simulink model "Q3"  (R2021b)
settings: Solver=ode45  StartTime=0.0  StopTime=30  RelTol=1e-3  EnableMultiTasking=on
undefined symbols (not defined in the file or in its folder): Hds, Hfs, Hus, V_s, Vs_nd
settings Model: Creator=ak  LastModifiedBy=user
settings SolverCC: AlgebraicLoopSolver=TrustRegion
settings DataIOCC: LimitDataPoints=on  SaveFormat=Array  ReturnWorkspaceOutputs=off
settings OptimizationCC: ExpressionDepthLimit=2147483647  LifeSpan=inf
settings DebuggingCC: UnderspecifiedInitializationDetection=Classic  MergeDetectMultiDrivingBlocksExec=none  SolverPrmCheckMsg=warning  StateNameClashWarn=warning  SFUnexpectedBacktrackingDiag=warning  SFNoUnconditionalDefaultTransitionDiag=warning  SFExecutionAtInitializationDiag=none  SFMachineParentedDataDiag=warning  ArithmeticOperatorsInVariantConditions=warning
settings HardwareCC: ProdBitPerPointer=32  ProdBitPerSizeT=32  ProdBitPerPtrDiffT=32  ProdLargestAtomicFloat=None  ProdIntDivRoundTo=Undefined  ProdEndianess=Unspecified  ProdWordSize=32  ProdHWDeviceType=32-bit Generic
settings ModelReferenceCC: PropagateSignalLabelsOutOfModel=off
settings SFSimCC: SimUseLocalCustomCode=off  CustomCodeUndefinedFunction=UseInterfaceOnly
settings RTWCC: RTWUseLocalCustomCode=off
settings CodeAppCC: StateflowObjectComments=on
settings GRTTargetCC: TargetLangStandard=C89/C90 (ANSI)
settings ConfigComp: CovMetricSettings=dw  CovSaveCumulativeToWorkspaceVar=on  CovSaveSingleToWorkspaceVar=on  CovExternalEMLEnable=off

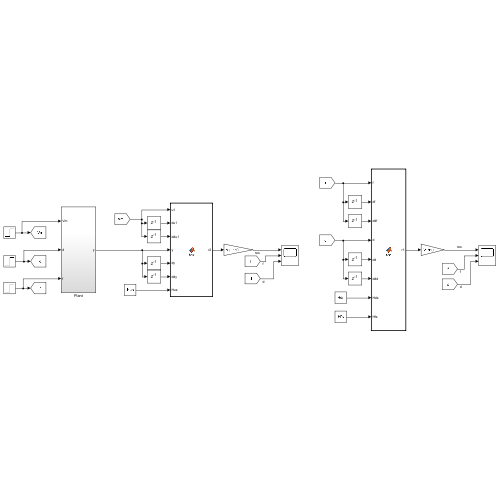
[thumbnail: Simulink's stored preview of the top-level diagram]
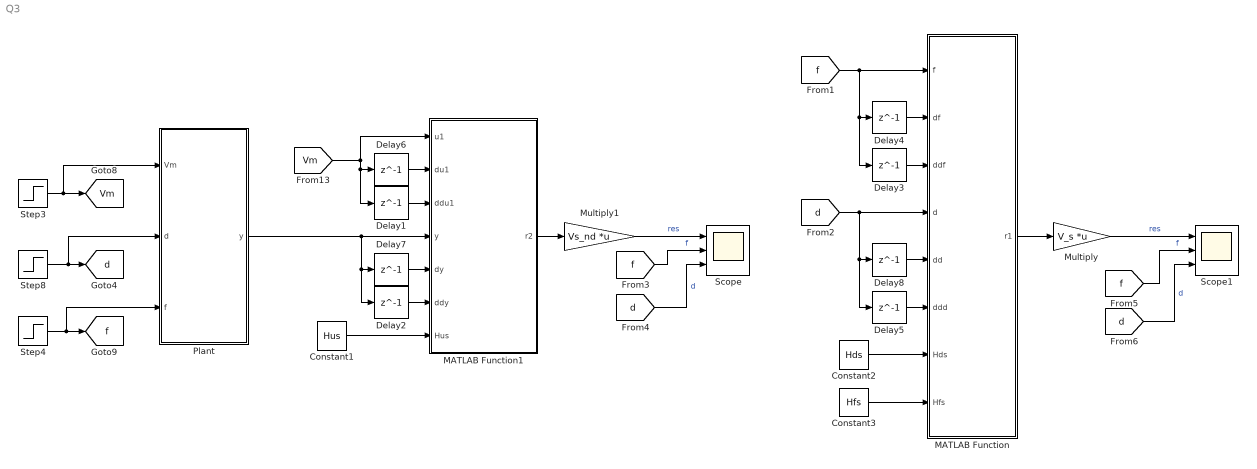
== system Q3 ==
  Constant1 : Constant  Value=Hus
  Constant2 : Constant  Value=Hds
  Constant3 : Constant  Value=Hfs
  Delay{1..8} (8 alike) : Delay  DelayLength=1  InitialCondition=0
  MATLAB Function : MATLAB Function  TreatAsAtomicUnit=on
  MATLAB Function1 : MATLAB Function  TreatAsAtomicUnit=on
  Multiply : Gain  Gain=V_s  Multiplication=Matrix(K*u)
  Multiply1 : Gain  Gain=Vs_nd  Multiplication=Matrix(K*u)
  Plant : Subsystem
  Scope : Scope  NumInputPorts=3
  Scope1 : Scope  NumInputPorts=3
  Step3 : Step  Time=0  After=2  SampleTime=0
  Step4 : Step  Time=2  After=2  SampleTime=0
  Step8 : Step  After=0.5  SampleTime=0
  tag scope: Vm=global, d=global, f=global
  wires:
  Step8/1 -> Plant/2(d), [d]
  Step4/1 -> Plant/3(f), [f]
  Step3/1 -> Plant/1(Vm), [Vm]
  Delay6/1 -> MATLAB Function1/2(du1)
  [Vm] -> MATLAB Function1/1(u1), Delay1/1, Delay6/1
  Plant/1(y) -> Delay2/1, Delay7/1, MATLAB Function1/4(y)
  MATLAB Function1/1(r2) -> Multiply1/1
  Constant1/1 -> MATLAB Function1/7(Hus)
  Delay7/1 -> MATLAB Function1/5(dy)
  Delay1/1 -> MATLAB Function1/3(ddu1)
  Delay2/1 -> MATLAB Function1/6(ddy)
  Multiply1/1 -> Scope/1  "res"
  [f] -> Scope/2  "f"
  [d] -> Scope/3  "d"
  [d] -> Scope1/3  "d"
  Multiply/1 -> Scope1/1  "res"
  [f] -> Delay3/1, Delay4/1, MATLAB Function/1(f)
  Constant3/1 -> MATLAB Function/8(Hfs)
  Constant2/1 -> MATLAB Function/7(Hds)
  MATLAB Function/1(r1) -> Multiply/1
  Delay4/1 -> MATLAB Function/2(df)
  Delay8/1 -> MATLAB Function/5(dd)
  [d] -> Delay5/1, Delay8/1, MATLAB Function/4(d)
  Delay5/1 -> MATLAB Function/6(ddd)
  [f] -> Scope1/2  "f"
  Delay3/1 -> MATLAB Function/3(ddf)

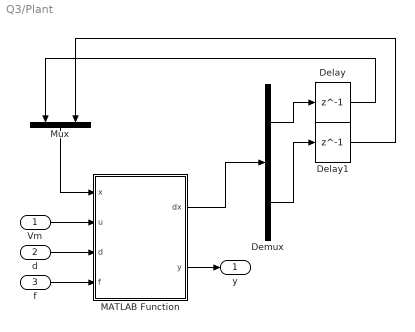
== system Q3/Plant ==
  Vm : Inport
  d : Inport  Port=2
  f : Inport  Port=3
  Delay : Delay  DelayLength=1  InputProcessing=Columns as channels (frame based)
  Delay1 : Delay  DelayLength=1  InputProcessing=Columns as channels (frame based)
  Demux : Demux  Outputs=2
  MATLAB Function : MATLAB Function  TreatAsAtomicUnit=on
  Mux : Mux  Inputs=2
  y : Outport
  wires:
  Vm/1 -> MATLAB Function/2(u)
  Mux/1 -> MATLAB Function/1(x)
  Demux/1 -> Delay/1
  Demux/2 -> Delay1/1
  Delay/1 -> Mux/1
  Delay1/1 -> Mux/2
  f/1 -> MATLAB Function/4(f)
  d/1 -> MATLAB Function/3(d)
  MATLAB Function/2(y) -> y/1
  MATLAB Function/1(dx) -> Demux/1

== matlab function Q3/MATLAB Function ==
  data: f input; r1 output; df input; ddf input; d input; dd input; ddd input; Hds input; Hfs input
function r1 = fcn(f,df,ddf,d,dd,ddd,Hds,Hfs)
d=[ddd;dd;d];
f=[ddf;df;f];
r1 = (Hds*d + Hfs*f);

== matlab function Q3/Plant/MATLAB Function ==
  data: x input; u input; dx output; d input; f input; y output
function [dx,y]  = plant(x,u,d,f)
% dx = zeros(2,1);
A = [0 1 ; -0.16 -1];
B = [0 ; 1];
C = [1 0];
Bd = [-0.1 ; 0];
Bf = [0.1 ; 0];
temp = A*x;
temp2 = B*u;
temp3 = Bd*d;
temp4 = Bf*f;
y=C*x;
dx = temp(:,1) + temp2(:,1) + temp3(:,1) + temp4(:,1);
end

== matlab function Q3/MATLAB Function1 ==
  data: u1 input; r2 output; du1 input; ddu1 input; y input; dy input; ddy input; Hus input
function r2 = fcn(u1,du1,ddu1,y,dy,ddy,Hus)
y=[ddy;dy;y];
u=[ddu1;du1;u1];
r2 = y-Hus*u;
